simulink model "GolfSwingZVCF"  (R2024a)
settings: Solver=VariableStepAuto  StartTime=0.0  StopTime=StopTime  MaxStep=0.001  RelTol=1e-3
PreLoadFcn:
  | cd(matlabdrive);
PostLoadFcn:
  | %run SCRIPT_mdlWksGenerate.m;
  | mdlWks=get_param('GolfSwingZVCF','ModelWorkspace');
  | mdlWks.DataSource = 'MAT-File';
  | mdlWks.FileName = 'ModelInputs.mat';
  | mdlWks.reload;
model workspace: external: MAT-File ModelInputsZVCF.mat (data not in the file)
undefined symbols (not defined in the file): JointTorqueHip, JointTorqueLElbow, JointTorqueLScap, JointTorqueLShoulder, JointTorqueLWrist, JointTorqueRElbow, JointTorqueRScap, JointTorqueRShoulder, JointTorqueRWrist, JointTorqueTorso, X, Y, Z
libraries: nesl_utility x286, sm_lib x176, matrix_library x11, simulink_extras x2
(part 1 of 9)
settings Model: Creator=dolso  LastModifiedBy=diete
settings SolverCC: MaxConsecutiveMinStep=20
settings DataIOCC: SaveOutput=off  DSMLogging=off
settings OptimizationCC: ReuseModelBlockBuffer=off
settings RTWCC: GPUComputeCapability=3.5
settings SimscapeCC: SimscapeLogLimitData=off

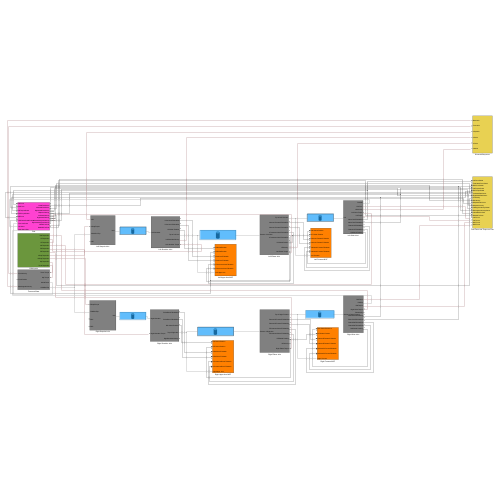
[thumbnail: Simulink's stored preview of the top-level diagram]
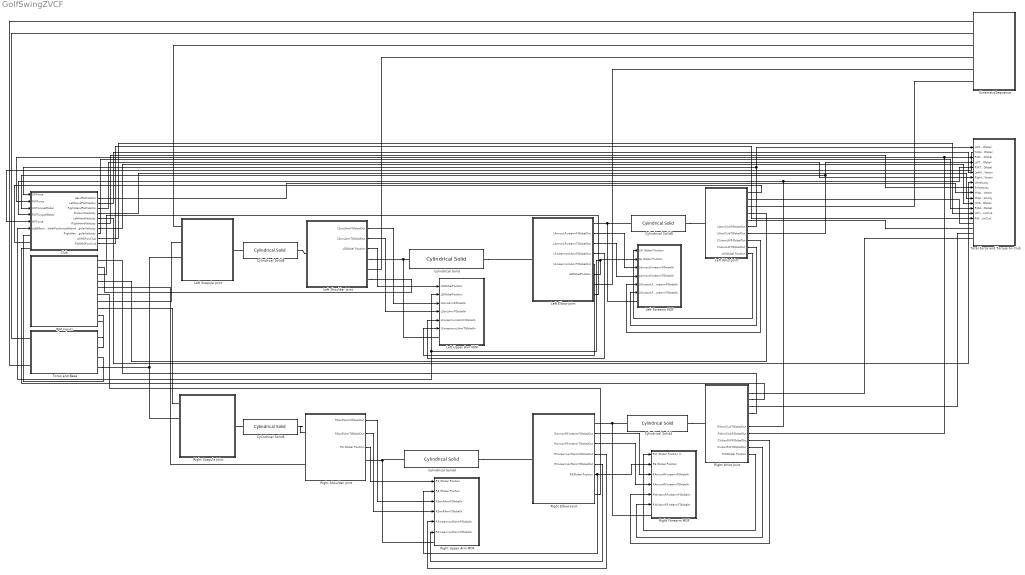
== system GolfSwingZVCF ==
  Club : Subsystem
  Cylindrical Solid : sm_lib/Body Elements/Cylindrical Solid  CylinderRadius=1.75  CylinderRadiusUnits=in  CylinderLength=12  CylinderLengthUnits=in  ExportEntireGeometry=off  InertiaType=CalculateFromGeometry  BasedOnType=Mass  Density=1000  DensityUnits=kg/m^3  Mass=5  MassUnits=lbm  CenterOfMass=[0 0 0]  CenterOfMassUnits=m  MomentsOfInertia=[1 1 1]  MomentsOfInertiaUnits=kg*m^2  ProductsOfInertia=[0 0 0]  ProductsOfInertiaUnits=kg*m^2  GraphicType=FromGeometry  MarkerShape=Sphere  MarkerSize=10  GraphicVisPropType=SimpleVisualProperties  GraphicDiffuseColor=[0.2 0.2 1.0]  GraphicOpacity=1.0  GraphicSpecularColor=[0.5 0.5 0.5 1.0]  GraphicAmbientColor=[0.15 0.15 0.15 1.0]  GraphicEmissiveColor=[0.0 0.0 0.0 1.0]  GraphicShininess=75  DoExposeReferenceFrame=off  SerializedFrames=<Frames><Frame><Id>Frame1</Id><Value><Name>Top of Left Arm</Name><Origin><Source>GeometricFeature</Source><FeatureName>top curve</FeatureName></Origin><PrimaryAxis><DefinedDirection>-X</DefinedDirection><Source>ReferenceFrame</Source><SourceDirection>+Z</SourceDirection><FeatureName></FeatureName></PrimaryAxis><SecondaryAxis><DefinedDirection>+Y</DefinedDirection><Source>ReferenceFrame</Source><SourceDirection>+X</SourceDirection><FeatureName></FeatureName></SecondaryAxis></Value></Frame><Frame><Id>Frame2</Id><Value><Name>Bottom of Left Arm</Name><Origin><Source>GeometricFeature</Source><FeatureName>bottom curve</FeatureName></Origin><PrimaryAxis><DefinedDirection>-X</DefinedDirection><Source>ReferenceFrame</Source><SourceDirection>+Z</SourceDirection><FeatureName></FeatureName></PrimaryAxis><SecondaryAxis><DefinedDirection>+Y</DefinedDirection><Source>ReferenceFrame</Source><SourceDirection>+X</SourceDirection><FeatureName></FeatureName></SecondaryAxis></Value></Frame></Frames>
  Cylindrical Solid3 : sm_lib/Body Elements/Cylindrical Solid  CylinderRadius=1.75  CylinderRadiusUnits=in  CylinderLength=12  CylinderLengthUnits=in  ExportEntireGeometry=off  InertiaType=CalculateFromGeometry  BasedOnType=Mass  Density=1000  DensityUnits=kg/m^3  Mass=5  MassUnits=lbm  CenterOfMass=[0 0 0]  CenterOfMassUnits=m  MomentsOfInertia=[1 1 1]  MomentsOfInertiaUnits=kg*m^2  ProductsOfInertia=[0 0 0]  ProductsOfInertiaUnits=kg*m^2  GraphicType=FromGeometry  MarkerShape=Sphere  MarkerSize=10  GraphicVisPropType=SimpleVisualProperties  GraphicDiffuseColor=[0.2 0.2 1.0]  GraphicOpacity=1.0  GraphicSpecularColor=[0.5 0.5 0.5 1.0]  GraphicAmbientColor=[0.15 0.15 0.15 1.0]  GraphicEmissiveColor=[0.0 0.0 0.0 1.0]  GraphicShininess=75  DoExposeReferenceFrame=off  SerializedFrames=<Frames><Frame><Id>Frame1</Id><Value><Name>Top of Right Arm</Name><Origin><Source>GeometricFeature</Source><FeatureName>top curve</FeatureName></Origin><PrimaryAxis><DefinedDirection>-X</DefinedDirection><Source>ReferenceFrame</Source><SourceDirection>+Z</SourceDirection><FeatureName></FeatureName></PrimaryAxis><SecondaryAxis><DefinedDirection>+Y</DefinedDirection><Source>ReferenceFrame</Source><SourceDirection>+X</SourceDirection><FeatureName></FeatureName></SecondaryAxis></Value></Frame><Frame><Id>Frame2</Id><Value><Name>Bottom of Right Arm</Name><Origin><Source>GeometricFeature</Source><FeatureName>bottom curve</FeatureName></Origin><PrimaryAxis><DefinedDirection>-X</DefinedDirection><Source>ReferenceFrame</Source><SourceDirection>+Z</SourceDirection><FeatureName></FeatureName></PrimaryAxis><SecondaryAxis><DefinedDirection>+Y</DefinedDirection><Source>ReferenceFrame</Source><SourceDirection>+X</SourceDirection><FeatureName></FeatureName></SecondaryAxis></Value></Frame></Frames>
  Cylindrical Solid4 : sm_lib/Body Elements/Cylindrical Solid  CylinderRadius=1.75  CylinderRadiusUnits=in  CylinderLength=14  CylinderLengthUnits=in  ExportEntireGeometry=off  InertiaType=CalculateFromGeometry  BasedOnType=Mass  Density=1000  DensityUnits=kg/m^3  Mass=5  MassUnits=lbm  CenterOfMass=[0 0 0]  CenterOfMassUnits=m  MomentsOfInertia=[1 1 1]  MomentsOfInertiaUnits=kg*m^2  ProductsOfInertia=[0 0 0]  ProductsOfInertiaUnits=kg*m^2  GraphicType=FromGeometry  MarkerShape=Sphere  MarkerSize=10  GraphicVisPropType=SimpleVisualProperties  GraphicDiffuseColor=[1.0 0.8 0.4]  GraphicOpacity=1.0  GraphicSpecularColor=[0.5 0.5 0.5 1.0]  GraphicAmbientColor=[0.15 0.15 0.15 1.0]  GraphicEmissiveColor=[0.0 0.0 0.0 1.0]  GraphicShininess=75  DoExposeReferenceFrame=off  SerializedFrames=<Frames><Frame><Id>Frame1</Id><Value><Name>Top of Right Forearm</Name><Origin><Source>GeometricFeature</Source><FeatureName>top curve</FeatureName></Origin><PrimaryAxis><DefinedDirection>-X</DefinedDirection><Source>ReferenceFrame</Source><SourceDirection>+Z</SourceDirection><FeatureName></FeatureName></PrimaryAxis><SecondaryAxis><DefinedDirection>+Y</DefinedDirection><Source>ReferenceFrame</Source><SourceDirection>+X</SourceDirection><FeatureName></FeatureName></SecondaryAxis></Value></Frame><Frame><Id>Frame2</Id><Value><Name>Bottom of Right Forearm</Name><Origin><Source>GeometricFeature</Source><FeatureName>bottom curve</FeatureName></Origin><PrimaryAxis><DefinedDirection>+X</DefinedDirection><Source>ReferenceFrame</Source><SourceDirection>-Z</SourceDirection><FeatureName></FeatureName></PrimaryAxis><SecondaryAxis><DefinedDirection>-Y</DefinedDirection><Source>ReferenceFrame</Source><SourceDirection>-X</SourceDirection><FeatureName></FeatureName></SecondaryAxis></Value></Frame></Frames>
  Cylindrical Solid5 : sm_lib/Body Elements/Cylindrical Solid  CylinderRadius=3  CylinderRadiusUnits=in  CylinderLength=10  CylinderLengthUnits=in  ExportEntireGeometry=off  InertiaType=CalculateFromGeometry  BasedOnType=Mass  Density=2000  DensityUnits=kg/m^3  Mass=10  MassUnits=kg  CenterOfMass=[0 0 0]  CenterOfMassUnits=m  MomentsOfInertia=[1 1 1]  MomentsOfInertiaUnits=kg*m^2  ProductsOfInertia=[0 0 0]  ProductsOfInertiaUnits=kg*m^2  GraphicType=FromGeometry  MarkerShape=Sphere  MarkerSize=10  GraphicVisPropType=SimpleVisualProperties  GraphicDiffuseColor=[0.2 0.2 1.0]  GraphicOpacity=1.0  GraphicSpecularColor=[0.5 0.5 0.5 1.0]  GraphicAmbientColor=[0.15 0.15 0.15 1.0]  GraphicEmissiveColor=[0.0 0.0 0.0 1.0]  GraphicShininess=75  DoExposeReferenceFrame=off  SerializedFrames=<Frames><Frame><Id>Frame1</Id><Value><Name>Hub</Name><Origin><Source>GeometricFeature</Source><FeatureName>top curve</FeatureName></Origin><PrimaryAxis><DefinedDirection>-X</DefinedDirection><Source>ReferenceFrame</Source><SourceDirection>-Z</SourceDirection><FeatureName></FeatureName></PrimaryAxis><SecondaryAxis><DefinedDirection>+Y</DefinedDirection><Source>ReferenceFrame</Source><SourceDirection>-X</SourceDirection><FeatureName></FeatureName></SecondaryAxis></Value></Frame><Frame><Id>Frame2</Id><Value><Name>Right Shoulder</Name><Origin><Source>GeometricFeature</Source><FeatureName>bottom curve</FeatureName></Origin><PrimaryAxis><DefinedDirection>-X</DefinedDirection><Source>ReferenceFrame</Source><SourceDirection>+Z</SourceDirection><FeatureName></FeatureName></PrimaryAxis><SecondaryAxis><DefinedDirection>+Y</DefinedDirection><Source>ReferenceFrame</Source><SourceDirection>+X</SourceDirection><FeatureName></FeatureName></SecondaryAxis></Value></Frame></Frames>
  Cylindrical Solid6 : sm_lib/Body Elements/Cylindrical Solid  CylinderRadius=3  CylinderRadiusUnits=in  CylinderLength=10  CylinderLengthUnits=in  ExportEntireGeometry=off  InertiaType=CalculateFromGeometry  BasedOnType=Mass  Density=2000  DensityUnits=kg/m^3  Mass=10  MassUnits=kg  CenterOfMass=[0 0 0]  CenterOfMassUnits=m  MomentsOfInertia=[1 1 1]  MomentsOfInertiaUnits=kg*m^2  ProductsOfInertia=[0 0 0]  ProductsOfInertiaUnits=kg*m^2  GraphicType=FromGeometry  MarkerShape=Sphere  MarkerSize=10  GraphicVisPropType=SimpleVisualProperties  GraphicDiffuseColor=[0.2 0.2 1.0]  GraphicOpacity=1.0  GraphicSpecularColor=[0.5 0.5 0.5 1.0]  GraphicAmbientColor=[0.15 0.15 0.15 1.0]  GraphicEmissiveColor=[0.0 0.0 0.0 1.0]  GraphicShininess=75  DoExposeReferenceFrame=off  SerializedFrames=<Frames><Frame><Id>Frame1</Id><Value><Name>Hub</Name><Origin><Source>GeometricFeature</Source><FeatureName>top curve</FeatureName></Origin><PrimaryAxis><DefinedDirection>-X</DefinedDirection><Source>ReferenceFrame</Source><SourceDirection>+Z</SourceDirection><FeatureName></FeatureName></PrimaryAxis><SecondaryAxis><DefinedDirection>+Y</DefinedDirection><Source>ReferenceFrame</Source><SourceDirection>+X</SourceDirection><FeatureName></FeatureName></SecondaryAxis></Value></Frame><Frame><Id>Frame2</Id><Value><Name>Left Shoulder</Name><Origin><Source>GeometricFeature</Source><FeatureName>bottom curve</FeatureName></Origin><PrimaryAxis><DefinedDirection>-X</DefinedDirection><Source>ReferenceFrame</Source><SourceDirection>+Z</SourceDirection><FeatureName></FeatureName></PrimaryAxis><SecondaryAxis><DefinedDirection>+Y</DefinedDirection><Source>ReferenceFrame</Source><SourceDirection>+X</SourceDirection><FeatureName></FeatureName></SecondaryAxis></Value></Frame></Frames>
  Cylindrical Solid8 : sm_lib/Body Elements/Cylindrical Solid  CylinderRadius=1.75  CylinderRadiusUnits=in  CylinderLength=14  CylinderLengthUnits=in  ExportEntireGeometry=off  InertiaType=CalculateFromGeometry  BasedOnType=Mass  Density=1000  DensityUnits=kg/m^3  Mass=5  MassUnits=lbm  CenterOfMass=[0 0 0]  CenterOfMassUnits=m  MomentsOfInertia=[1 1 1]  MomentsOfInertiaUnits=kg*m^2  ProductsOfInertia=[0 0 0]  ProductsOfInertiaUnits=kg*m^2  GraphicType=FromGeometry  MarkerShape=Sphere  MarkerSize=10  GraphicVisPropType=SimpleVisualProperties  GraphicDiffuseColor=[1.0 0.8 0.4]  GraphicOpacity=1.0  GraphicSpecularColor=[0.5 0.5 0.5 1.0]  GraphicAmbientColor=[0.15 0.15 0.15 1.0]  GraphicEmissiveColor=[0.0 0.0 0.0 1.0]  GraphicShininess=75  DoExposeReferenceFrame=off  SerializedFrames=<Frames><Frame><Id>Frame1</Id><Value><Name>Top of Left Forearm</Name><Origin><Source>GeometricFeature</Source><FeatureName>top curve</FeatureName></Origin><PrimaryAxis><DefinedDirection>-X</DefinedDirection><Source>ReferenceFrame</Source><SourceDirection>+Z</SourceDirection><FeatureName></FeatureName></PrimaryAxis><SecondaryAxis><DefinedDirection>+Y</DefinedDirection><Source>ReferenceFrame</Source><SourceDirection>+X</SourceDirection><FeatureName></FeatureName></SecondaryAxis></Value></Frame><Frame><Id>Frame2</Id><Value><Name>Left Wrist</Name><Origin><Source>GeometricFeature</Source><FeatureName>bottom curve</FeatureName></Origin><PrimaryAxis><DefinedDirection>-X</DefinedDirection><Source>ReferenceFrame</Source><SourceDirection>+Z</SourceDirection><FeatureName></FeatureName></PrimaryAxis><SecondaryAxis><DefinedDirection>+Y</DefinedDirection><Source>ReferenceFrame</Source><SourceDirection>+X</SourceDirection><FeatureName></FeatureName></SecondaryAxis></Value></Frame></Frames>
  KinematicSequence : Subsystem
  Left Elbow Joint : Subsystem
      settings: PortSchema="{\"entries\":[{\"content\":{\"sides\":[{\"content\":{\"connectorIds\":[\"LConn1\"]},\"type\":\"ConnectorPlacement.EquallySpacedRectSide\",\"uuid\":\"0d2dc99c-eb11-4109-9a2b-17505465b565\"},{\"content\":{\"connectorIds\":[\"RConn1\",\"Out1\",\"Out2\",\"Out3\",\"Out4\",\"Out5\",\"RConn2\",\"RConn3\"],\"side\":\"RIGHT\"},\"type\":\"ConnectorPlacement.EquallySpacedRectSide\",\"uuid\":\"6ecd8be0-02d3-4d37-82cf-97f4ae3a7b62\"},{\"content\":{\"side\":\"TOP\"},\"type\":\"ConnectorPlacement.EquallySpacedRectSide\",\"uuid\":\"fc24cd9c-45b2-4b41-afed-7be465f4fbe9\"}]},\"type\":\"ConnectorPlacement.EquallySpacedConnector\",\"uuid\":\"efc9acae-06dd-440e-9911-40f18f1b9237\"}],\"packageUris\":[\"http://schema.mathworks.com/mf0/Connector/R2020b\"],\"version\":\"1.0\"}"
  Left Forearm MOF : Subsystem
  Left Scapula Joint : Subsystem
  Left Shoulder Joint : Subsystem
  Left Upper Arm MOF : Subsystem
  Left Wrist Joint : Subsystem
      settings: PortSchema="{\"entries\":[{\"content\":{\"sides\":[{\"content\":{\"connectorIds\":[\"LConn1\"]},\"type\":\"ConnectorPlacement.EquallySpacedRectSide\",\"uuid\":\"73e94019-3378-46e9-afbe-4641b41dde8c\"},{\"content\":{\"connectorIds\":[\"RConn1\",\"RConn2\",\"RConn3\",\"RConn4\",\"RConn5\",\"Out1\",\"Out2\",\"Out3\",\"Out4\",\"Out5\"],\"side\":\"RIGHT\"},\"type\":\"ConnectorPlacement.EquallySpacedRectSide\",\"uuid\":\"33c81984-e3a3-4521-b427-302dfd6552c2\"},{\"content\":{\"side\":\"TOP\"},\"type\":\"ConnectorPlacement.EquallySpacedRectSide\",\"uuid\":\"972c8ae3-eaf7-4328-abd2-22356629bb46\"}]},\"type\":\"ConnectorPlacement.EquallySpacedConnector\",\"uuid\":\"c2ac63b4-2c7d-42b0-87d6-e1245c4ebe36\"}],\"packageUris\":[\"http://schema.mathworks.com/mf0/Connector/R2020b\"],\"version\":\"1.0\"}"
  RJM Inputs : Subsystem
  Right Elbow Joint : Subsystem
      settings: PortSchema="{\"entries\":[{\"content\":{\"sides\":[{\"content\":{\"connectorIds\":[\"LConn1\"]},\"type\":\"ConnectorPlacement.EquallySpacedRectSide\",\"uuid\":\"0d2dc99c-eb11-4109-9a2b-17505465b565\"},{\"content\":{\"connectorIds\":[\"RConn1\",\"Out1\",\"Out2\",\"Out3\",\"Out4\",\"Out5\",\"RConn2\",\"RConn3\"],\"side\":\"RIGHT\"},\"type\":\"ConnectorPlacement.EquallySpacedRectSide\",\"uuid\":\"6ecd8be0-02d3-4d37-82cf-97f4ae3a7b62\"},{\"content\":{\"side\":\"TOP\"},\"type\":\"ConnectorPlacement.EquallySpacedRectSide\",\"uuid\":\"fc24cd9c-45b2-4b41-afed-7be465f4fbe9\"}]},\"type\":\"ConnectorPlacement.EquallySpacedConnector\",\"uuid\":\"efc9acae-06dd-440e-9911-40f18f1b9237\"}],\"packageUris\":[\"http://schema.mathworks.com/mf0/Connector/R2020b\"],\"version\":\"1.0\"}"
  Right Forearm MOF : Subsystem
  Right Scapula Joint : Subsystem
  Right Shoulder Joint : Subsystem
  Right Upper Arm MOF : Subsystem
  Right Wrist Joint : Subsystem
      settings: PortSchema="{\"entries\":[{\"content\":{\"sides\":[{\"content\":{\"connectorIds\":[\"LConn1\"]},\"type\":\"ConnectorPlacement.EquallySpacedRectSide\",\"uuid\":\"9550879f-a378-40e1-8a95-adbfddbfedc1\"},{\"content\":{\"connectorIds\":[\"RConn1\",\"RConn2\",\"RConn3\",\"RConn4\",\"RConn5\",\"Out1\",\"Out2\",\"Out3\",\"Out4\",\"Out5\"],\"side\":\"RIGHT\"},\"type\":\"ConnectorPlacement.EquallySpacedRectSide\",\"uuid\":\"54c31fca-6ae0-4a69-a999-2c488770e2d4\"},{\"content\":{\"side\":\"TOP\"},\"type\":\"ConnectorPlacement.EquallySpacedRectSide\",\"uuid\":\"5a050cdf-0b22-482f-bf5e-43478f01f3c5\"}]},\"type\":\"ConnectorPlacement.EquallySpacedConnector\",\"uuid\":\"8ff0b9f4-f1d2-4dc5-a94c-e903db69229e\"}],\"packageUris\":[\"http://schema.mathworks.com/mf0/Connector/R2020b\"],\"version\":\"1.0\"}"
  Torso and Base : Subsystem
  Total Force and Torque on Club : Subsystem
      settings: PortSchema="{\"entries\":[{\"content\":{\"sides\":[{\"content\":{\"connectorIds\":[\"In1\",\"Out1\",\"In2\",\"In3\",\"In4\",\"In5\",\"In6\",\"In7\",\"In8\",\"In9\",\"In10\",\"In11\",\"In12\",\"In13\",\"In14\",\"LConn1\",\"LConn2\",\"LConn3\",\"LConn4\"]},\"type\":\"ConnectorPlacement.EquallySpacedRectSide\",\"uuid\":\"e49b0733-7688-4c06-bf4b-d9bdb9b271ad\"},{\"content\":{\"side\":\"RIGHT\"},\"type\":\"ConnectorPlacement.EquallySpacedRectSide\",\"uuid\":\"ff6a27b2-fdee-4bae-bdac-9c564ad2a9e4\"},{\"content\":{\"side\":\"TOP\"},\"type\":\"ConnectorPlacement.EquallySpacedRectSide\",\"uuid\":\"d6331d59-6720-42ef-8b86-9cce389eab9b\"}]},\"type\":\"ConnectorPlacement.EquallySpacedConnector\",\"uuid\":\"5f69422c-1f90-45af-9a45-06188f2db8f9\"}],\"packageUris\":[\"http://schema.mathworks.com/mf0/Connector/R2020b\"],\"version\":\"1.0\"}"
  wires:
  Club/1(HandPathVector) -> Total Force and Torque on Club/9(MidpointPathVector)
  Total Force and Torque on Club/1(TotalHandForceGlobal) -> Club/5(MPForce)
  Left Wrist Joint/1(LWonClubFGlobalOut) -> Total Force and Torque on Club/1(LWForceGlobal), Club/1(LWForce)
  Left Wrist Joint/2(LWonClubTGlobalOut) -> Total Force and Torque on Club/3(LWTorqueGlobal), Club/3(LWTorqueGlobal)
  Right Wrist Joint/2(RWonClubFGlobalOut) -> Total Force and Torque on Club/2(RWForceGlobal), Club/2(RWForce)
  Right Wrist Joint/1(RWonClubTGlobalOut) -> Total Force and Torque on Club/4(RWTorqueGlobal), Club/4(RWTorqueGlobal)
  Club/2(LeftHandPathVector) -> Total Force and Torque on Club/5(LeftHandPathVector)
  Club/3(RightHandPathVector) -> Total Force and Torque on Club/6(RightHandPathVector)
  Right Elbow Joint/5(REGlobal Position) -> Right Forearm MOF/2(RE Global Position), Right Upper Arm MOF/2(RE Global Position)
  Left Shoulder Joint/3(LSGlobal Position) -> Left Upper Arm MOF/1(LSGlobalPosition)
  Left Wrist Joint/5(LWGlobal Position) -> Left Forearm MOF/1(LW Global Position)
  Right Shoulder Joint/3(RS Global Position) -> Right Upper Arm MOF/1(RS Global Position)
  Right Wrist Joint/5(RWGlobal Position) -> Right Forearm MOF/1(RW Global Position In)
  Left Shoulder Joint/1(LSonLArmFGlobalOut) -> Left Upper Arm MOF/3(LSonLArmFGlobalIn)
  Left Shoulder Joint/2(LSonLArmTGlobalOut) -> Left Upper Arm MOF/4(LSonLArmTGlobalIn)
  Left Elbow Joint/3(LForearmonLArmFGlobalOut) -> Left Upper Arm MOF/5(LForearmonLArmFGlobalIn)
  Left Elbow Joint/4(LForearmonLArmTGlobalOut) -> Left Upper Arm MOF/6(LForearmonLArmTGlobalIn)
  Right Shoulder Joint/2(RSonRArmTGlobalOut) -> Right Upper Arm MOF/4(RSonRArmTGlobalIn)
  Right Shoulder Joint/1(RSonRArmFGlobalOut) -> Right Upper Arm MOF/3(RSonRArmFGlobalIn)
  Right Elbow Joint/3(RForearmonRArmFGlobalOut) -> Right Upper Arm MOF/5(RForearmonRArmFGlobalIn)
  Right Elbow Joint/4(RForearmonRArmTGlobalOut) -> Right Upper Arm MOF/6(RForearmonRArmTGlobalIn)
  Left Elbow Joint/1(LArmonLForearmFGlobalOut) -> Left Forearm MOF/3(LArmonLForearmFGlobalIn)
  Left Elbow Joint/2(LArmonLForearmTGlobalOut) -> Left Forearm MOF/4(LArmonLForearmTGlobalIn)
  Left Wrist Joint/3(ClubonLWFGlobalOut) -> Left Forearm MOF/5(LWristonLForearmFGlobalIn)
  Left Wrist Joint/4(ClubonLWTGlobalOut) -> Left Forearm MOF/6(LWristonLForearmTGlobalIn)
  Right Elbow Joint/1(RArmonRForearmFGlobalOut) -> Right Forearm MOF/3(RArmonRForearmFGlobalIn)
  Right Elbow Joint/2(RArmonRForearmTGlobalOut) -> Right Forearm MOF/4(RArmonRForearmTGlobalIn)
  Right Wrist Joint/3(ClubonRWFGlobalOut) -> Right Forearm MOF/5(RWristonRForearmFGlobalIn)
  Right Wrist Joint/4(ClubonRWTGlobalOut) -> Right Forearm MOF/6(RWristonRForearmTGlobalIn)
  Club/4(MidpointVelocity) -> Total Force and Torque on Club/10(MidpointVelocity)
  Club/5(LeftHandVelocity) -> Total Force and Torque on Club/7(LHVelocity)
  Club/6(RightHandVelocity) -> Total Force and Torque on Club/8(RHVelocity)
  Club/7(LeftHandAngularVelocity) -> Total Force and Torque on Club/11(LWAngularVelocityGlobal)
  Club/8(RightHandAngularVelocity) -> Total Force and Torque on Club/12(RWAngularVelocityGlobal)
  Club/9(LWMOFonClub) -> Total Force and Torque on Club/13(LWristMOFonClub)
  Club/10(RW0MOFonClub) -> Total Force and Torque on Club/14(RWMOFonClub)
  Left Elbow Joint/5(LEGlobalPosition) -> Left Upper Arm MOF/2(LEGlobalPosition), Club/6(LeftElbowGlobalPosition), Left Forearm MOF/2(LE Global Position)
  connections:
  Cylindrical Solid6/RConn1 -- Left Shoulder Joint/LConn1
  Right Upper Arm MOF/LConn1 -- Cylindrical Solid3/LConn1 -- Right Shoulder Joint/RConn1
  Cylindrical Solid5/RConn1 -- Right Shoulder Joint/LConn1
  Left Shoulder Joint/RConn1 -- Left Upper Arm MOF/LConn1 -- Cylindrical Solid/LConn1
  Cylindrical Solid4/LConn1 -- Right Forearm MOF/LConn1 -- Right Elbow Joint/RConn1
  Cylindrical Solid3/RConn1 -- Right Elbow Joint/LConn1
  Cylindrical Solid4/RConn1 -- Right Wrist Joint/LConn1
  Left Elbow Joint/RConn3 -- RJM Inputs/RConn3
  RJM Inputs/RConn4 -- Left Wrist Joint/RConn4
  Left Shoulder Joint/RConn3 -- RJM Inputs/RConn2
  Right Wrist Joint/RConn1 -- Total Force and Torque on Club/LConn4
  Right Wrist Joint/RConn2 -- Club/LConn3
  Club/LConn1 -- Torso and Base/RConn3
  Club/LConn2 -- Left Wrist Joint/RConn1
  KinematicSequence/LConn5 -- Left Elbow Joint/RConn2
  KinematicSequence/LConn4 -- Left Shoulder Joint/RConn2
  KinematicSequence/LConn6 -- Left Wrist Joint/RConn3
  Torso and Base/RConn4 -- Right Scapula Joint/LConn2 -- Left Scapula Joint/LConn3
  Torso and Base/LConn3 -- KinematicSequence/LConn1
  Torso and Base/LConn1 -- KinematicSequence/LConn2
  Torso and Base/RConn2 -- RJM Inputs/RConn9
  Torso and Base/RConn1 -- RJM Inputs/RConn10
  Right Shoulder Joint/LConn2 -- RJM Inputs/RConn5
  Right Wrist Joint/RConn4 -- RJM Inputs/RConn1
  Right Elbow Joint/RConn3 -- RJM Inputs/RConn6
  Right Wrist Joint/RConn3 -- Total Force and Torque on Club/LConn3
  Total Force and Torque on Club/LConn1 -- Left Wrist Joint/RConn2
  Cylindrical Solid8/LConn1 -- Left Forearm MOF/LConn1 -- Left Elbow Joint/RConn1
  Cylindrical Solid8/RConn1 -- Left Wrist Joint/LConn1
  Cylindrical Solid/RConn1 -- Left Elbow Joint/LConn1
  Left Scapula Joint/LConn1 -- KinematicSequence/LConn3
  Cylindrical Solid6/LConn1 -- Left Scapula Joint/RConn1
  Left Scapula Joint/LConn2 -- RJM Inputs/RConn7
  RJM Inputs/RConn8 -- Right Scapula Joint/LConn1
  Cylindrical Solid5/LConn1 -- Right Scapula Joint/RConn1
  Left Wrist Joint/RConn5 -- Total Force and Torque on Club/LConn2

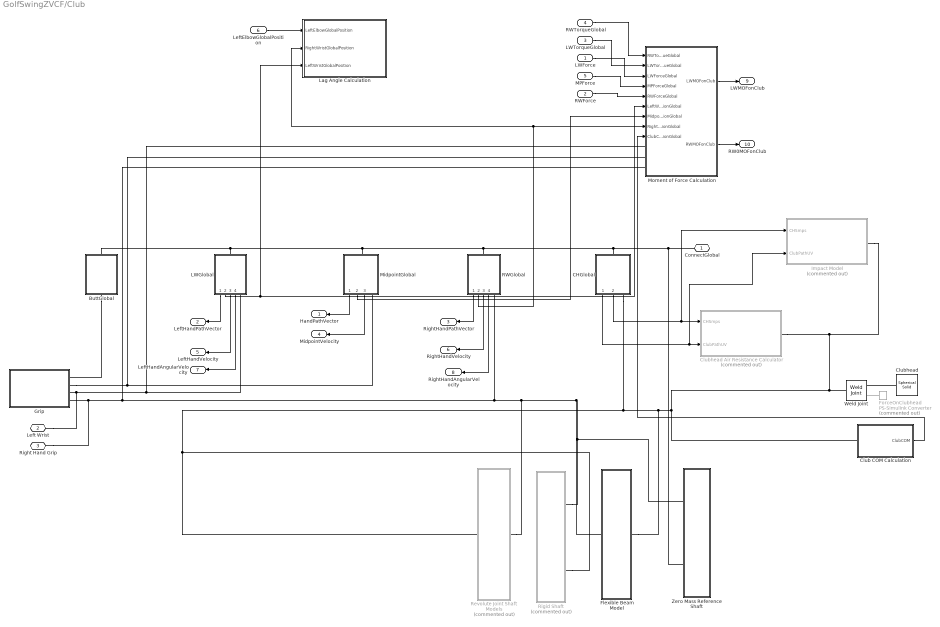
== system GolfSwingZVCF/Club ==
  LWForce : Inport
  RWForce : Inport  Port=2
  LWTorqueGlobal : Inport  Port=3
  RWTorqueGlobal : Inport  Port=4
  MPForce : Inport  Port=5
  LeftElbowGlobalPosition : Inport  Port=6
  ButtGlobal : Subsystem
  CHGlobal : Subsystem
  Club COM Calculation : Subsystem
  Clubhead : sm_lib/Body Elements/Spherical Solid  SphereRadius=ClubheadRadius  SphereRadiusUnits=in  ExportEntireGeometry=off  InertiaType=CalculateFromGeometry  BasedOnType=Mass  Density=500  DensityUnits=kg/m^3  Mass=0.25  MassUnits=kg  CenterOfMass=[0 0 0]  CenterOfMassUnits=m  MomentsOfInertia=[1 1 1]  MomentsOfInertiaUnits=kg*m^2  ProductsOfInertia=[0 0 0]  ProductsOfInertiaUnits=kg*m^2  GraphicType=FromGeometry  MarkerShape=Sphere  MarkerSize=10  GraphicVisPropType=SimpleVisualProperties  GraphicDiffuseColor=[0.0 0.0 0.0]  GraphicOpacity=1.0  GraphicSpecularColor=[0.5 0.5 0.5 1.0]  GraphicAmbientColor=[0.15 0.15 0.15 1.0]  GraphicEmissiveColor=[0.0 0.0 0.0 1.0]  GraphicShininess=75  DoExposeReferenceFrame=on  SerializedFrames=<Frames/>
  Clubhead Air Resistance Calculator : Subsystem  Commented=on
  Flexible Beam Model : Subsystem
  ForceOnClubhead : nesl_utility/PS-Simulink Converter  Commented=on  PhysicalDomain=network_engine_domain  SubClassName=ps_output  LeftPortType=input  RightPortType=output  PseudoPeriodic=off  Frequencies=[]  VectorFormat=1-D array  Unit=inherit  AffineConversion=off
  Grip : Subsystem
  Impact Model : Subsystem  Commented=on
  LWGlobal : Subsystem
  Lag Angle Calculation : Subsystem
  MidpointGlobal : Subsystem
  Moment of Force Calculation : Subsystem
  RWGlobal : Subsystem
  Revolute Joint Shaft Models : Subsystem  Commented=on
  Rigid Shaft : Subsystem  Commented=on
  Weld Joint : sm_lib/Joints/Weld Joint  JointMode=Normal  CompositeWrenchDir=BaseOnFollower  CompositeWrenchFrame=BaseFrame  SenseConstraintForce=off  SenseConstraintTorque=off  SenseTotalForce=on  SenseTotalTorque=off
  Zero Mass Reference Shaft : Subsystem
  ConnectGlobal : PMIOPort  Side=Left
  Left Wrist : PMIOPort  Port=2  Side=Left
  Right Hand Grip : PMIOPort  Port=3  Side=Left
  HandPathVector : Outport
  LeftHandPathVector : Outport  Port=2
  RightHandPathVector : Outport  Port=3
  MidpointVelocity : Outport  Port=4
  LeftHandVelocity : Outport  Port=5
  RightHandVelocity : Outport  Port=6
  LeftHandAngularVelocity : Outport  Port=7
  RightHandAngularVelocity : Outport  Port=8
  LWMOFonClub : Outport  Port=9
  RW0MOFonClub : Outport  Port=10
  wires:
  MidpointGlobal/1(HandPathVector) -> HandPathVector/1
  RWGlobal/1(RightHandPathVector) -> RightHandPathVector/1
  LWGlobal/1(LeftHandPathVector) -> LeftHandPathVector/1
  LWForce/1 -> Moment of Force Calculation/3(LWForceGlobal)
  MPForce/1 -> Moment of Force Calculation/4(MPForceGlobal)
  RWForce/1 -> Moment of Force Calculation/5(RWForceGlobal)
  MidpointGlobal/2(MidHandPosition) -> Moment of Force Calculation/7(MidpointPositionGlobal)
  RWGlobal/2(RightHandPosition) -> Lag Angle Calculation/2(RightWristGlobalPosition), Moment of Force Calculation/8(RightWristPositionGlobal)
  Club COM Calculation/1(ClubCOM) -> Moment of Force Calculation/9(ClubCOMPositionGlobal)
  LWTorqueGlobal/1 -> Moment of Force Calculation/2(LWTorqueGlobal)
  RWTorqueGlobal/1 -> Moment of Force Calculation/1(RWTorqueGlobal)
  CHGlobal/1(ClubPathUV) -> Impact Model/2(ClubPathUV), Clubhead Air Resistance Calculator/2(ClubPathUV)
  CHGlobal/2(CHSMPS) -> Impact Model/1(CHSmps), Clubhead Air Resistance Calculator/1(CHSmps)
  MidpointGlobal/3(MidHandVelocity) -> MidpointVelocity/1
  LWGlobal/3(LHVelocity) -> LeftHandVelocity/1
  RWGlobal/3(RHVelocity) -> RightHandVelocity/1
  LWGlobal/4(LeftWristGlobalAV) -> LeftHandAngularVelocity/1
  RWGlobal/4(RightWristGlobalAV) -> RightHandAngularVelocity/1
  Moment of Force Calculation/1(LWMOFonClub) -> LWMOFonClub/1
  Moment of Force Calculation/2(RWMOFonClub) -> RW0MOFonClub/1
  LWGlobal/2(LeftHandPosition) -> Lag Angle Calculation/3(LeftWristGlobalPosition), Moment of Force Calculation/6(LeftWristPositionGlobal)
  LeftElbowGlobalPosition/1 -> Lag Angle Calculation/1(LeftElbowGlobalPosition)
  connections:
  LWGlobal/RConn1 -- Left Wrist/RConn1 -- Grip/RConn3 -- Moment of Force Calculation/LConn1
  Grip/RConn2 -- Moment of Force Calculation/LConn2 -- MidpointGlobal/RConn1
  ButtGlobal/RConn1 -- Grip/RConn1
  RWGlobal/LConn1 -- ButtGlobal/LConn1 -- LWGlobal/LConn1 -- MidpointGlobal/LConn1 -- ConnectGlobal/RConn1 -- Zero Mass Reference Shaft/RConn2 -- CHGlobal/LConn1
  CHGlobal/RConn1 -- Rigid Shaft/RConn2 -- Revolute Joint Shaft Models/LConn1 -- Flexible Beam Model/RConn1 -- Club COM Calculation/LConn1 -- Clubhead Air Resistance Calculator/RConn1 -- Impact Model/RConn1 -- Weld Joint/LConn1
  ForceOnClubhead/LConn1 -- Weld Joint/RConn2
  Clubhead/RConn1 -- Weld Joint/RConn1
  Zero Mass Reference Shaft/RConn1 -- Grip/RConn4 -- Right Hand Grip/RConn1 -- Moment of Force Calculation/LConn3 -- RWGlobal/RConn1 -- Revolute Joint Shaft Models/RConn1 -- Flexible Beam Model/LConn1 -- Rigid Shaft/RConn1

== system GolfSwingZVCF/KinematicSequence ==
  BaseAV : nesl_utility/PS-Simulink Converter  PhysicalDomain=network_engine_domain  SubClassName=ps_output  LeftPortType=input  RightPortType=output  PseudoPeriodic=off  Frequencies=[]  VectorFormat=inherit  Unit=deg/s  AffineConversion=off
  ChestAV : Sum
  ClubhandleAV : Sum
  LEAV : nesl_utility/PS-Simulink Converter  PhysicalDomain=network_engine_domain  SubClassName=ps_output  LeftPortType=input  RightPortType=output  PseudoPeriodic=off  Frequencies=[]  VectorFormat=inherit  Unit=deg/s  AffineConversion=off
  LSAV : nesl_utility/PS-Simulink Converter  PhysicalDomain=network_engine_domain  SubClassName=ps_output  LeftPortType=input  RightPortType=output  PseudoPeriodic=off  Frequencies=[]  VectorFormat=inherit  Unit=deg/s  AffineConversion=off
  LScapAV : nesl_utility/PS-Simulink Converter  PhysicalDomain=network_engine_domain  SubClassName=ps_output  LeftPortType=input  RightPortType=output  PseudoPeriodic=off  Frequencies=[]  VectorFormat=inherit  Unit=deg/s  AffineConversion=off
  LWAV : nesl_utility/PS-Simulink Converter  PhysicalDomain=network_engine_domain  SubClassName=ps_output  LeftPortType=input  RightPortType=output  PseudoPeriodic=off  Frequencies=[]  VectorFormat=inherit  Unit=deg/s  AffineConversion=off
  LeftForearmAV : Sum
  LeftScapulaAV : Sum
  LeftUpperArmAV : Sum
  TorsoAV : nesl_utility/PS-Simulink Converter  PhysicalDomain=network_engine_domain  SubClassName=ps_output  LeftPortType=input  RightPortType=output  PseudoPeriodic=off  Frequencies=[]  VectorFormat=inherit  Unit=deg/s  AffineConversion=off
  BaseAVIn : PMIOPort  Side=Left
  TorsoAVIn : PMIOPort  Port=2  Side=Left
  LSapAVIn : PMIOPort  Port=3  Side=Left
  LSAVIn : PMIOPort  Port=4  Side=Left
  LEAVIn : PMIOPort  Port=5  Side=Left
  LWAVIn : PMIOPort  Port=6  Side=Left
  wires:
  LeftUpperArmAV/1 -> LeftForearmAV/1  "LUpperArmAV"
  ChestAV/1 -> LeftScapulaAV/1  "ChestAV"
  LeftScapulaAV/1 -> LeftUpperArmAV/1  "LScapAV"
  LeftForearmAV/1 -> ClubhandleAV/1  "LForearmAV"
  LEAV/1 -> LeftForearmAV/2
  LWAV/1 -> ClubhandleAV/2
  LScapAV/1 -> LeftScapulaAV/2
  BaseAV/1 -> ChestAV/1  "BaseAV"
  TorsoAV/1 -> ChestAV/2
  LSAV/1 -> LeftUpperArmAV/2
  connections:
  LEAVIn/RConn1 -- LEAV/LConn1
  TorsoAVIn/RConn1 -- TorsoAV/LConn1
  LSAVIn/RConn1 -- LSAV/LConn1
  LSapAVIn/RConn1 -- LScapAV/LConn1
  BaseAVIn/RConn1 -- BaseAV/LConn1
  LWAVIn/RConn1 -- LWAV/LConn1

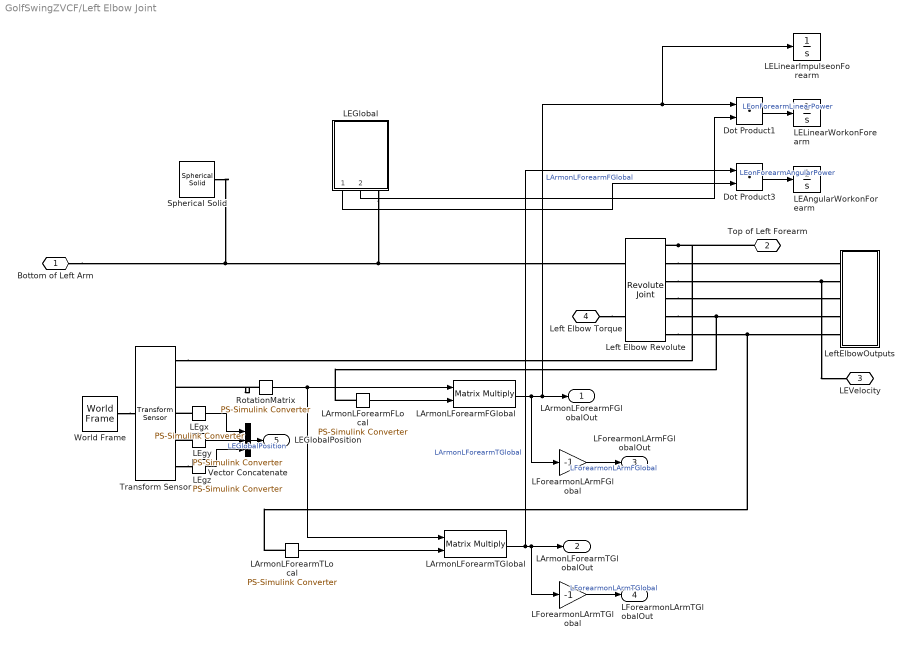
== system GolfSwingZVCF/Left Elbow Joint ==
  Dot Product1 : DotProduct  OutDataTypeStr=Inherit: Inherit via internal rule
  Dot Product3 : DotProduct  OutDataTypeStr=Inherit: Inherit via internal rule
  LArmonLForearmFGlobal : Product  Multiplication=Matrix(*)
  LArmonLForearmFLocal : nesl_utility/PS-Simulink Converter  PhysicalDomain=network_engine_domain  SubClassName=ps_output  LeftPortType=input  RightPortType=output  PseudoPeriodic=off  Frequencies=[]  VectorFormat=1-D array  Unit=inherit  AffineConversion=off
  LArmonLForearmTGlobal : Product  Multiplication=Matrix(*)
  LArmonLForearmTLocal : nesl_utility/PS-Simulink Converter  PhysicalDomain=network_engine_domain  SubClassName=ps_output  LeftPortType=input  RightPortType=output  PseudoPeriodic=off  Frequencies=[]  VectorFormat=1-D array  Unit=inherit  AffineConversion=off
  LEAngularWorkonForearm : Integrator
  LEGlobal : Subsystem
  LELinearImpulseonForearm : Integrator
  LELinearWorkonForearm : Integrator
  LEgx : nesl_utility/PS-Simulink Converter  PhysicalDomain=network_engine_domain  SubClassName=ps_output  LeftPortType=input  RightPortType=output  PseudoPeriodic=off  Frequencies=[]  VectorFormat=1-D array  Unit=inherit  AffineConversion=off
  LEgy : nesl_utility/PS-Simulink Converter  PhysicalDomain=network_engine_domain  SubClassName=ps_output  LeftPortType=input  RightPortType=output  PseudoPeriodic=off  Frequencies=[]  VectorFormat=1-D array  Unit=inherit  AffineConversion=off
  LEgz : nesl_utility/PS-Simulink Converter  PhysicalDomain=network_engine_domain  SubClassName=ps_output  LeftPortType=input  RightPortType=output  PseudoPeriodic=off  Frequencies=[]  VectorFormat=1-D array  Unit=inherit  AffineConversion=off
  LForearmonLArmFGlobal : Gain  Gain=-1
  LForearmonLArmTGlobal : Gain  Gain=-1
  Left Elbow Revolute : sm_lib/Joints/Revolute Joint  JointMode=Normal  CompositeWrenchDir=BaseOnFollower  CompositeWrenchFrame=FollowerFrame  SenseConstraintForce=off  SenseConstraintTorque=off  SenseTotalForce=on  SenseTotalTorque=on  PositionTargetSpecify=on  PositionTargetPriority=High  PositionTargetValue=LElbowStartPosition  PositionTargetValueUnits=deg  VelocityTargetSpecify=on  VelocityTargetPriority=High  VelocityTargetValue=LElbowStartVelocity  VelocityTargetValueUnits=deg/s  EquilibriumPosition=0  EquilibriumPositionUnits=deg  SpringStiffness=0  SpringStiffnessUnits=N*m/deg  DampingCoefficient=0  DampingCoefficientUnits=N*m/(deg/s)  LowerLimitSpecify=off  LowerLimitBound=-20  LowerLimitBoundUnits=deg  LowerLimitStiffness=1  LowerLimitStiffnessUnits=N*m/deg  LowerLimitDamping=0  LowerLimitDampingUnits=N*m/(deg/s)  LowerLimitTransitionRegionWidth=0.1  LowerLimitTransitionRegionWidthUnits=deg  UpperLimitSpecify=off  UpperLimitBound=20  UpperLimitBoundUnits=deg  UpperLimitStiffness=1e3  UpperLimitStiffnessUnits=N*m/deg  UpperLimitDamping=10  UpperLimitDampingUnits=N*m/(deg/s)  UpperLimitTransitionRegionWidth=0.1  UpperLimitTransitionRegionWidthUnits=deg  TorqueActuationMode=InputTorque  MotionActuationMode=ComputedMotion  SensePosition=on  SenseVelocity=on  SenseAcceleration=on  SenseTorqueForce=off  SenseLowerLimitTorqueForce=off  SenseUpperLimitTorqueForce=off
      settings: LogSimulationData=on
  LeftElbowOutputs : Subsystem
  RotationMatrix : nesl_utility/PS-Simulink Converter  PhysicalDomain=network_engine_domain  SubClassName=ps_output  LeftPortType=input  RightPortType=output  PseudoPeriodic=off  Frequencies=[]  VectorFormat=1-D array  Unit=inherit  AffineConversion=off
  Spherical Solid : sm_lib/Body Elements/Spherical Solid  SphereRadius=1.75  SphereRadiusUnits=in  ExportEntireGeometry=off  InertiaType=CalculateFromGeometry  BasedOnType=Density  Density=0  DensityUnits=kg/m^3  Mass=1  MassUnits=kg  CenterOfMass=[0 0 0]  CenterOfMassUnits=m  MomentsOfInertia=[1 1 1]  MomentsOfInertiaUnits=kg*m^2  ProductsOfInertia=[0 0 0]  ProductsOfInertiaUnits=kg*m^2  GraphicType=FromGeometry  MarkerShape=Sphere  MarkerSize=10  GraphicVisPropType=SimpleVisualProperties  GraphicDiffuseColor=[1.0 0.8 0.4]  GraphicOpacity=1  GraphicSpecularColor=[0.5 0.5 0.5 1.0]  GraphicAmbientColor=[0.15 0.15 0.15 1.0]  GraphicEmissiveColor=[0.0 0.0 0.0 1.0]  GraphicShininess=75  DoExposeReferenceFrame=on  SerializedFrames=<Frames/>
  Transform Sensor : sm_lib/Frames and Transforms/Transform Sensor  MeasurementFrame=World  RotationSequence=XYX  SenseAngle=off  SenseAxis=off  SenseQ=off  SenseR=on  SenseRotationSequence=off  SenseOmegaX=off  SenseOmegaY=off  SenseOmegaZ=off  SenseOmega=off  SenseQDot=off  SenseRDot=off  SenseRotationSequenceDot=off  SenseAlphaX=off  SenseAlphaY=off  SenseAlphaZ=off  SenseAlpha=off  SenseQDDot=off  SenseRDDot=off  SenseX=on  SenseY=on  SenseZ=on  SenseXYZ=off  SenseRad=off  SenseAzim=off  SenseDist=off  SenseInc=off  SenseXDot=off  SenseYDot=off  SenseZDot=off  SenseXYZDot=off  SenseRadDot=off  SenseAzimDot=off  SenseDistDot=off  SenseIncDot=off  SenseXDDot=off  SenseYDDot=off  SenseZDDot=off  SenseXYZDDot=off  SenseRadDDot=off  SenseAzimDDot=off  SenseDistDDot=off  SenseIncDDot=off
  Vector Concatenate : Concatenate  NumInputs=3
  World Frame : sm_lib/Frames and Transforms/World Frame
  Bottom of Left Arm : PMIOPort  Side=Left
  Top of Left Forearm : PMIOPort  Port=2  Side=Right
  LEVelocity : PMIOPort  Port=3  Side=Right
  Left Elbow Torque : PMIOPort  Port=4  Side=Right
  LArmonLForearmFGlobalOut : Outport
  LArmonLForearmTGlobalOut : Outport  Port=2
  LForearmonLArmFGlobalOut : Outport  Port=3
  LForearmonLArmTGlobalOut : Outport  Port=4
  LEGlobalPosition : Outport  Port=5
  wires:
  LArmonLForearmTLocal/1 -> LArmonLForearmTGlobal/2
  LForearmonLArmTGlobal/1 -> LForearmonLArmTGlobalOut/1  "LForearmonLArmTGlobal"
  RotationMatrix/1 -> LArmonLForearmFGlobal/1, LArmonLForearmTGlobal/1
  LArmonLForearmFLocal/1 -> LArmonLForearmFGlobal/2
  LForearmonLArmFGlobal/1 -> LForearmonLArmFGlobalOut/1  "LForearmonLArmFGlobal"
  LArmonLForearmTGlobal/1 -> LArmonLForearmTGlobalOut/1, LForearmonLArmTGlobal/1, Dot Product3/1  "LArmonLForearmTGlobal"
  LEgx/1 -> Vector Concatenate/1
  LEgz/1 -> Vector Concatenate/3
  Vector Concatenate/1 -> LEGlobalPosition/1  "LEGlobalPosition"
  LEgy/1 -> Vector Concatenate/2
  Dot Product3/1 -> LEAngularWorkonForearm/1  "LEonForearmAngularPower"
  Dot Product1/1 -> LELinearWorkonForearm/1  "LEonForearmLinearPower"
  LEGlobal/1(LeftElbowGlobalAV) -> Dot Product3/2
  LEGlobal/2(LeftElbowGlobalVelocity) -> Dot Product1/2
  LArmonLForearmFGlobal/1 -> LForearmonLArmFGlobal/1, LELinearImpulseonForearm/1, Dot Product1/1, LArmonLForearmFGlobalOut/1  "LArmonLForearmFGlobal"
  connections:
  Left Elbow Revolute/RConn4 -- LeftElbowOutputs/LConn3
  Left Elbow Revolute/RConn2 -- LeftElbowOutputs/LConn1
  Left Elbow Revolute/RConn1 -- Top of Left Forearm/RConn1 -- Transform Sensor/RConn1
  Left Elbow Revolute/RConn6 -- LArmonLForearmTLocal/LConn1 -- LeftElbowOutputs/LConn5
  Left Elbow Revolute/RConn3 -- LEVelocity/RConn1 -- LeftElbowOutputs/LConn2
  Spherical Solid/RConn1 -- LEGlobal/RConn1 -- Left Elbow Revolute/LConn1 -- Bottom of Left Arm/RConn1
  Left Elbow Torque/RConn1 -- Left Elbow Revolute/LConn2
  Left Elbow Revolute/RConn5 -- LArmonLForearmFLocal/LConn1 -- LeftElbowOutputs/LConn4
  World Frame/RConn1 -- Transform Sensor/LConn1
  RotationMatrix/LConn1 -- Transform Sensor/RConn2
  LEgx/LConn1 -- Transform Sensor/RConn3
  Transform Sensor/RConn5 -- LEgz/LConn1
  LEgy/LConn1 -- Transform Sensor/RConn4

== system GolfSwingZVCF/Left Forearm MOF ==
  LW Global Position : Inport
  LE Global Position : Inport  Port=2
  LArmonLForearmFGlobalIn : Inport  Port=3
  LArmonLForearmTGlobalIn : Inport  Port=4
  LWristonLForearmFGlobalIn : Inport  Port=5
  LWristonLForearmTGlobalIn : Inport  Port=6
  LEAngularImpulseonForearm : Integrator
  LElbowonLForearmMOFGlobal : matrix_library/Cross Product
  LElbowonLForearmMOFLocal : Product  Multiplication=Matrix(*)
  LFCOM : sm_lib/Body Elements/Inertia Sensor  SensorExtent=BodyGroup  SpanWeldJoints=off  ExcludeGroundedBodies=off  MeasurementFrame=World  SenseMass=off  SenseCenterOfMass=on  SenseInertiaMatrix=off  SenseCenteredInertiaMatrix=off  SensePrincipalInertiaMatrix=off  SenseRotationMatrix=off  GraphicType=None  PrincipalInertiaFrameSize=20  GraphicVisPropType=SimpleVisualProperties  GraphicDiffuseColor=[0.5 0.5 0.5]  GraphicOpacity=1  GraphicSpecularColor=[0.5 0.5 0.5 1.0]  GraphicAmbientColor=[0.15 0.15 0.15 1.0]  GraphicEmissiveColor=[0.0 0.0 0.0 1.0]  GraphicShininess=75
  LWristonLForearmMOFGlobal : matrix_library/Cross Product
  LWristonLForearmMOFLocal : Product  Multiplication=Matrix(*)
  Left Forearm COM : nesl_utility/PS-Simulink Converter  PhysicalDomain=network_engine_domain  SubClassName=ps_output  LeftPortType=input  RightPortType=output  PseudoPeriodic=off  Frequencies=[]  VectorFormat=1-D array  Unit=inherit  AffineConversion=off
  R Vector Elbow Force on Left Forearm : Sum  Inputs=-+
  R Vector Wrist Force on Left Forearm : Sum  Inputs=-+
  RotationTransformLeftHand : nesl_utility/PS-Simulink Converter  PhysicalDomain=network_engine_domain  SubClassName=ps_output  LeftPortType=input  RightPortType=output  PseudoPeriodic=off  Frequencies=[]  VectorFormat=1-D array  Unit=inherit  AffineConversion=off
  SumofMomentsLEonLForearm : Sum
  SumofMomentsLForearmLocal : Product  Multiplication=Matrix(*)
  SumofMomentsLeftForearmGlobal : Sum  Inputs=++++
  Transform Sensor : sm_lib/Frames and Transforms/Transform Sensor  MeasurementFrame=World  RotationSequence=XYX  SenseAngle=off  SenseAxis=off  SenseQ=off  SenseR=on  SenseRotationSequence=off  SenseOmegaX=off  SenseOmegaY=off  SenseOmegaZ=off  SenseOmega=off  SenseQDot=off  SenseRDot=off  SenseRotationSequenceDot=off  SenseAlphaX=off  SenseAlphaY=off  SenseAlphaZ=off  SenseAlpha=off  SenseQDDot=off  SenseRDDot=off  SenseX=off  SenseY=off  SenseZ=off  SenseXYZ=off  SenseRad=off  SenseAzim=off  SenseDist=off  SenseInc=off  SenseXDot=off  SenseYDot=off  SenseZDot=off  SenseXYZDot=off  SenseRadDot=off  SenseAzimDot=off  SenseDistDot=off  SenseIncDot=off  SenseXDDot=off  SenseYDDot=off  SenseZDDot=off  SenseXYZDDot=off  SenseRadDDot=off  SenseAzimDDot=off  SenseDistDDot=off  SenseIncDDot=off
  World Frame : sm_lib/Frames and Transforms/World Frame
  Left Forearm : PMIOPort  Side=Left
  wires:
  Left Forearm COM/1 -> R Vector Elbow Force on Left Forearm/1, R Vector Wrist Force on Left Forearm/1  "LeftForearmCOM"
  LE Global Position/1 -> R Vector Elbow Force on Left Forearm/2
  LW Global Position/1 -> R Vector Wrist Force on Left Forearm/2
  R Vector Elbow Force on Left Forearm/1 -> LElbowonLForearmMOFGlobal/1
  LArmonLForearmFGlobalIn/1 -> LElbowonLForearmMOFGlobal/2
  R Vector Wrist Force on Left Forearm/1 -> LWristonLForearmMOFGlobal/1
  LWristonLForearmTGlobalIn/1 -> SumofMomentsLeftForearmGlobal/4
  LWristonLForearmFGlobalIn/1 -> LWristonLForearmMOFGlobal/2
  SumofMomentsLeftForearmGlobal/1 -> SumofMomentsLForearmLocal/2  "SumofMomentsLeftForearmGlobal"
  LWristonLForearmMOFGlobal/1 -> LWristonLForearmMOFLocal/2, SumofMomentsLeftForearmGlobal/2  "LWristonLForearmMOFGlobal"
  RotationTransformLeftHand/1 -> SumofMomentsLForearmLocal/1, LWristonLForearmMOFLocal/1, LElbowonLForearmMOFLocal/1
  LElbowonLForearmMOFGlobal/1 -> SumofMomentsLEonLForearm/2, LElbowonLForearmMOFLocal/2, SumofMomentsLeftForearmGlobal/1  "LElbowonLForearmMOFGlobal"
  SumofMomentsLEonLForearm/1 -> LEAngularImpulseonForearm/1  "SumofMomentsLEonLForearm"
  LArmonLForearmTGlobalIn/1 -> SumofMomentsLEonLForearm/1, SumofMomentsLeftForearmGlobal/3
  connections:
  LFCOM/LConn1 -- Transform Sensor/LConn1 -- Left Forearm/RConn1
  LFCOM/RConn1 -- Left Forearm COM/LConn1
  Transform Sensor/RConn1 -- World Frame/RConn1
  RotationTransformLeftHand/LConn1 -- Transform Sensor/RConn2

== system GolfSwingZVCF/Left Scapula Joint ==
  LSOutput : Subsystem
  Left Scapula : sm_lib/Joints/Revolute Joint  JointMode=Normal  CompositeWrenchDir=BaseOnFollower  CompositeWrenchFrame=FollowerFrame  SenseConstraintForce=off  SenseConstraintTorque=off  SenseTotalForce=on  SenseTotalTorque=on  PositionTargetSpecify=on  PositionTargetPriority=High  PositionTargetValue=LScapStartPosition  PositionTargetValueUnits=deg  VelocityTargetSpecify=on  VelocityTargetPriority=High  VelocityTargetValue=LScapStartVelocity  VelocityTargetValueUnits=deg/s  EquilibriumPosition=0  EquilibriumPositionUnits=deg  SpringStiffness=0  SpringStiffnessUnits=N*m/deg  DampingCoefficient=0  DampingCoefficientUnits=N*m/(deg/s)  LowerLimitSpecify=off  LowerLimitBound=-90  LowerLimitBoundUnits=deg  LowerLimitStiffness=1e4  LowerLimitStiffnessUnits=N*m/deg  LowerLimitDamping=10  LowerLimitDampingUnits=N*m/(deg/s)  LowerLimitTransitionRegionWidth=0.1  LowerLimitTransitionRegionWidthUnits=deg  UpperLimitSpecify=off  UpperLimitBound=90  UpperLimitBoundUnits=deg  UpperLimitStiffness=1e4  UpperLimitStiffnessUnits=N*m/deg  UpperLimitDamping=10  UpperLimitDampingUnits=N*m/(deg/s)  UpperLimitTransitionRegionWidth=0.1  UpperLimitTransitionRegionWidthUnits=deg  TorqueActuationMode=InputTorque  MotionActuationMode=ComputedMotion  SensePosition=on  SenseVelocity=on  SenseAcceleration=off  SenseTorqueForce=off  SenseLowerLimitTorqueForce=off  SenseUpperLimitTorqueForce=off
  LSV : PMIOPort  Side=Left
  LScapTorque : PMIOPort  Port=2  Side=Left
  COM Rod Top : PMIOPort  Port=3  Side=Left
  LSP : PMIOPort  Port=4  Side=Left
  Hub : PMIOPort  Port=5  Side=Right
  connections:
  Left Scapula/LConn1 -- COM Rod Top/RConn1
  Left Scapula/RConn5 -- LSOutput/LConn3
  Left Scapula/RConn4 -- LSOutput/LConn4
  Hub/RConn1 -- Left Scapula/RConn1
  Left Scapula/RConn2 -- LSP/RConn1 -- LSOutput/LConn2
  LSOutput/LConn1 -- LSV/RConn1 -- Left Scapula/RConn3
  Left Scapula/LConn2 -- LScapTorque/RConn1
